simulink model "testblock_103_Harness_test1"  (R2022b)
settings: Solver=FixedStepAuto  StartTime=0.0  StopTime=10  FixedStep=0.01  RelTol=1e-3
libraries: SignalEditorBlockLib x1
settings Model: Creator=Brigosha_Guest  LastModifiedBy=Brigosha_Guest

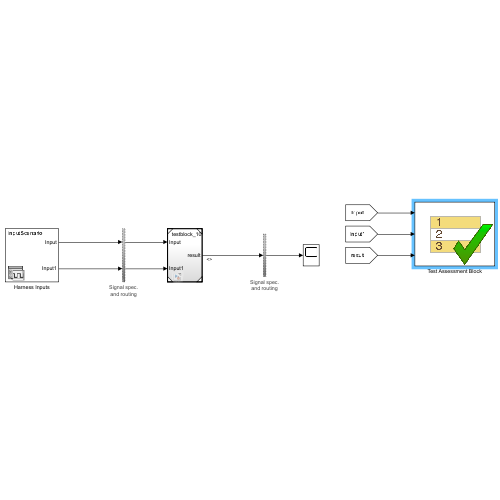
[thumbnail: Simulink's stored preview of the top-level diagram]
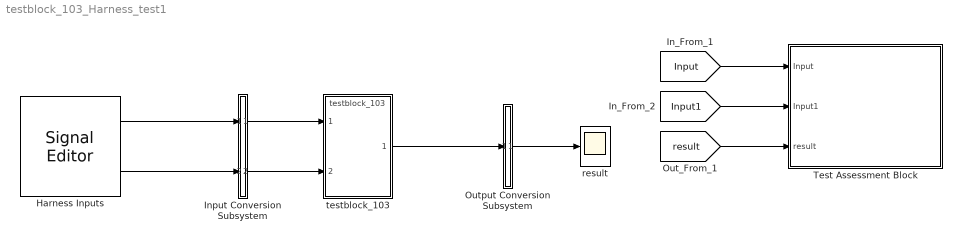
== system testblock_103_Harness_test1 ==
  Harness Inputs : SignalEditorBlockLib/Signal Editor  FileName=C:\matlab_prog\test_harness_model\testblock_103_Harness_test1_HarnessInputs.mat  ActiveScenario=InputScenario  ActiveSignal=Input  IsBus=off  OutputBusObjectStr=Bus: BusObject  SampleTime=0.01  Interpolate=off  ZeroCross=off  OutputAfterFinalValue=Setting to zero  Unit=inherit  PreserveSignalName=on
  Input Conversion Subsystem : Subsystem  Tag=__SLT_ICS__  Description=|
      | Signal spec.
      | and routing
      settings: AttributesFormatString=%<Description>
  Output Conversion Subsystem : Subsystem  Tag=__SLT_OCS__  Description=|
      | Signal spec.
      | and routing
      settings: AttributesFormatString=%<Description>
  Test Assessment Block : Test Sequence  Tag=__SLT_ASMT__  TreatAsAtomicUnit=on
  result : Scope
  testblock_103 : ModelReference  ModelNameDialog=testblock_103  SimulationMode=Normal  ModelReferenceVersion=1.5
  wires:
  [Input] -> Test Assessment Block/1(Input)
  [Input1] -> Test Assessment Block/2(Input1)
  [result] -> Test Assessment Block/3(result)
  Harness Inputs/1 -> Input Conversion Subsystem/1(Inport_1)
  Harness Inputs/2 -> Input Conversion Subsystem/2(Inport_2)
  Output Conversion Subsystem/1(Outport_1) -> result/1
  Input Conversion Subsystem/1(Outport_1) -> testblock_103/1
  Input Conversion Subsystem/2(Outport_2) -> testblock_103/2
  testblock_103/1 -> Output Conversion Subsystem/1(Inport_1)

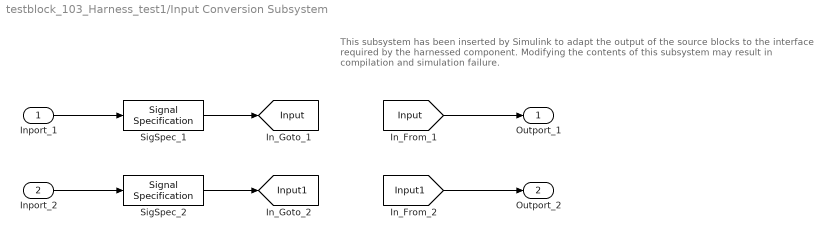
== system testblock_103_Harness_test1/Input Conversion Subsystem ==
  note: This subsystem has been inserted by Simulink to adapt the output of the source blocks to the interface required by the harnessed component.
      |  Modifying the contents of this subsystem may result in compilation and simulation failure.
  Inport_1 : Inport
  Inport_2 : Inport  Port=2
  SigSpec_1 : SignalSpecification  OutDataTypeStr=double  Dimensions=[1]  SampleTime=0.01
  SigSpec_2 : SignalSpecification  OutDataTypeStr=double  Dimensions=[1]  SampleTime=0.01
  Outport_1 : Outport
  Outport_2 : Outport  Port=2
  tag scope: Input1=global, Input=global
  wires:
  [Input] -> Outport_1/1
  SigSpec_1/1 -> [Input]
  Inport_1/1 -> SigSpec_1/1
  [Input1] -> Outport_2/1
  SigSpec_2/1 -> [Input1]
  Inport_2/1 -> SigSpec_2/1

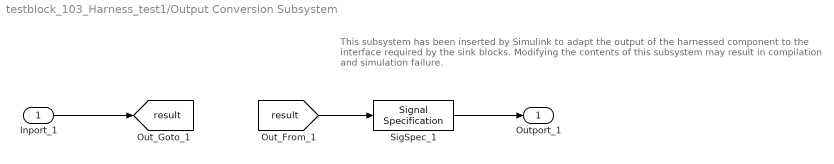
== system testblock_103_Harness_test1/Output Conversion Subsystem ==
  note: This subsystem has been inserted by Simulink to adapt the output of the harnessed component to the interface required by the sink blocks.
      |  Modifying the contents of this subsystem may result in compilation and simulation failure.
  Inport_1 : Inport
  SigSpec_1 : SignalSpecification  OutDataTypeStr=double  Dimensions=[1]  SampleTime=0.01
  Outport_1 : Outport
  tag scope: result=global
  wires:
  Inport_1/1 -> [result]
  [result] -> SigSpec_1/1
  SigSpec_1/1 -> Outport_1/1

== stateflow chart testblock_103_Harness_test1/Test Assessment Block ==
  state Run
    state step_1_1
    state step_1_2
    (default) -> (junction 22)
    Run -> (junction 22)
    (junction 22) -> (junction 23) [order 1] : [t < 5
        | ]
    (junction 23) -> step_1_1 [order 1] : [~in(Run.step_1_1)]
    (junction 23) -> (junction 26) [order 2]
    (junction 31) -> (junction 32)
    (junction 32) -> step_1_2 [order 1] : [~in(Run.step_1_2)]
    (junction 32) -> (junction 35) [order 2]
    (junction 22) -> (junction 31) [order 2]
  (default) -> Run
  data: Input input double size=[1]; Input1 input double size=[1]; result input double size=[1]
